simulink subsystem "station1"  (R2024b)
settings: Solver=VariableStepAuto  StartTime=0.0  StopTime=10.0  RelTol=1e-3
undefined symbols (not defined in the file): DiscIntNeverNeededParam, DPL1ph, h, Half, R3, ResistanceM, Rt4, simetran, Ts, Zm
libraries: fl_lib x215, ee_lib x97, nesl_utility x43, spsThreePhaseHarmonicFilterLib x21, simulink x7, spsThreePhaseSeriesRLCLoadLib x7, spsThreePhaseBreakerLib x7
(part 3 of 6)

== system station1/Filters 60Hz5 ==
  note: 60 Hz filters 4*150 Mvars @ 500 kV
  note: High-pass
      | damped filter
  note: Tuned filters
  note: Capacitor banks
  s : Inport
  11th 150 Mvar Q=100 : spsThreePhaseHarmonicFilterLib/Three-Phase Harmonic Filter  Commented=on  LConnTagsString=A|B|C  FilterType=Single-tuned  FilterConnection=Y (grounded)  ParNom=[500e3 60]  Qc=150e6/4  Fr=[11*60]  Frd=[11*60 13*60]  Q=100  Measurements=None
      settings: AttributesFormatString=\n
      settings: LibrarySourceBlock=|
      | sps_lib/Passives/Three-Phase
      | Harmonic Filter
  "13th 150 Mvar Q=100 " : spsThreePhaseHarmonicFilterLib/Three-Phase Harmonic Filter  Commented=on  LConnTagsString=A|B|C  FilterType=Single-tuned  FilterConnection=Y (grounded)  ParNom=[500e3 60]  Qc=150e6/4  Fr=[13*60]  Frd=[11*60 13*60]  Q=100  Measurements=None
      settings: AttributesFormatString=\n
      settings: LibrarySourceBlock=|
      | sps_lib/Passives/Three-Phase
      | Harmonic Filter
  150 Mvar : spsThreePhaseSeriesRLCLoadLib/Three-Phase Series RLC Load  Commented=on  LConnTagsString=A|B|C  Configuration=Y (grounded)  NominalVoltage=500e3  Vabc=[1e3 1e3 1e3]  Vabcp=[1e3 1e3 1e3]  NominalFrequency=60  UnbalancedPower=off  ActivePower=0  InductivePower=0  CapacitivePower=150e6/4  Pabc=[10e3 9e3 11e3]  QLabc=[100 90 110]  QCabc=[100 90 110]  Pabcp=[10e3 9e3 11e3]  QLabcp=[100 90 110]  QCabcp=[100 90 110]  Measurements=None  LoadType=constant Z
  24th 150 Mvar Q=3 : spsThreePhaseHarmonicFilterLib/Three-Phase Harmonic Filter  Commented=on  LConnTagsString=A|B|C  FilterType=High-pass  FilterConnection=Y (grounded)  ParNom=[500e3 60]  Qc=150e6/4  Fr=[24*60]  Frd=[11*60 13*60]  Q=3  Measurements=None
      settings: AttributesFormatString=\n
      settings: LibrarySourceBlock=|
      | sps_lib/Passives/Three-Phase
      | Harmonic Filter
  Circuit Breaker (Three-Phase) : ee_lib/Switches & Breakers/Circuit Breaker (Three-Phase)  R_closed=0.001 Ohm  G_open=1e-6 1/Ohm  threshold=0.5 V  breaker_behavior=ee.enum.switches.breakerBehavior.zeroCrossingEnable
      settings: InternalSimscapePortConfiguration="{\"Bottom\":[],\"Left\":[{\"id\":\"vT\",\"label\":\"vT\",\"type\":\"input\"},{\"id\":\"N1\",\"label\":\"~1\",\"type\":\"foundation.electrical.three_phase\"}],\"Right\":[{\"id\":\"N2\",\"label\":\"~2\",\"type\":\"foundation.electrical.three_phase\"}],\"Top\":[]}"
  Constant : Constant
  Electrical Reference : fl_lib/Electrical/Electrical Elements/Electrical Reference
  High-pass filter : Subsystem  mask(Three-Phase Harmonic Filter){FilterType=High-pass, FilterConnection=Y (grounded), ParNom=[500e3 60], Qc=150e6/4, Fr=[5*60], Frd=[24*60], Q=3}
      mask prompts: FilterType "Type of filter:"; FilterConnection "Filter connection:"; ParNom "Nominal L-L voltage and frequency  [Vn(Vrms) fn(Hz)]:"; Qc "Nominal reactive power (var):"; Fr "Tuning frequency (Hz)"; Frd "Tuning frequencies [ Fr1 (Hz)   Fr2 (Hz) ]"; Q "Quality factor (Q):"
      mask help:
      | Implements a three-phase harmonic filter.
      | The filter is built up from passive RLC components. Their values are computed using the specified  nominal reactive power, tuning frequency (ies) and quality factor.
      mask init: same as station1/Filters 60Hz1/High-pass filter
      mask Help: helpview(psbhelp);
      mask TypeOptions FilterType: Single-tuned | Double-tuned | High-pass | C-type High-pass
      mask Callback FilterType: %powericon('ThreePhaseHarmonicFilterCback',gcb);
      mask TypeOptions FilterConnection: Y (grounded) | Y (floating) | Y (neutral) | Delta
      mask Callback FilterConnection: %powericon('ThreePhaseHarmonicFilterCback',gcb);
      mask Display:
      | plot(12,0,88,95)
      | plot(C1_xo+cx0,C1_yo+cy0,C1_xo+cx1,C1_yo+cy1,C1_xo+cx2,C1_yo+cy2,C1_xo+cx3,C1_yo+cy3)
      | plot(L1_xo+lx0,L1_yo+ly0,L1_xo+lx1,L1_yo+ly1,L1_xo+lx2,L1_yo+ly2,L1_xo+lx3,L1_yo+ly3,L1_xo+lx4,L1_yo+ly4)
      | plot(R1_xo+rx0,R1_yo+ry0,R1_xo+rx1,R1_yo+ry1,R1_xo+rx2,R1_yo+ry2)
      | plot(C2_xo+cx0,C2_yo+cy0,C2_xo+cx1,C2_yo+cy1,C2_xo+cx2,C2_yo+cy2,C2_xo+cx3,C2_yo+cy3)
      | plot(L2_xo+lx0,L2_yo+ly0,L2_xo+lx1,L2_yo+ly1,L2_xo+lx2,L2_yo+ly2,L2_xo+lx3,L2_yo+ly3,L2_xo+lx4,L2_yo+ly4)
      | plot(s1x,s1y,s2x,s2y,s3x,s3y,s4x,s4y)
      | plot(g_xo+gx1,g_yo+gy1,g_xo+gx2,g_yo+gy2,g_xo+gx3,g_yo+gy3,g_xo+gx4,g_yo+gy4)
  Simulink-PS Converter : nesl_utility/Simulink-PS Converter  PhysicalDomain=network_engine_domain  SubClassName=ps_input  LeftPortType=input  RightPortType=output  PseudoPeriodic=off  Frequencies=[]  NoiseDistribution=none  NoiseParameters=[]  Unit=1  AffineConversion=off  FilteringAndDerivatives=provide  SimscapeFilterOrder=1  InputFilterTimeConstant=0.001  UdotUserProvided=0
  Sum : Sum  Inputs=|-+
  Three-Phase Breaker : spsThreePhaseBreakerLib/Three-Phase Breaker  Commented=on  InitialState=open  SwitchA=on  SwitchB=on  SwitchC=on  SwitchTimes=[1.5]  External=on  BreakerResistance=0.001  SnubberResistance=1e6  SnubberCapacitance=inf  Measurements=None
  Wye-Connected Load : ee_lib/Passive/RLC Assemblies/Wye-Connected Load  port_option=ee.enum.threePhasePort.composite  parameterization=ee.enum.rlc.parameterization.ratedpower  component_structure=ee.enum.rlc.structure.R  component_structure_PQ=ee.enum.rlc.structure.C  R=1 Ohm  L=1e-3 H  C=1e-6 F  VRated=500e3 V  FRated=60 Hz  P=1e3 W  Qpos=1e2 A*V  Qneg=-150e6/4 A*V  R_parasitic=1e-6 Ohm  G_parasitic=1e-6 1/Ohm  R_parasitic_PQ=0 Ohm  G_parasitic_PQ=1e-6 1/Ohm  Vmag0=500e3 V  Vang0=0 deg  Freq0=60 Hz  IL_specify=off  IL_priority=High  IL=[0, 0, 0] A  IL_nominal_specify=off  IL_nominal_value=1  IL_nominal_unit=A  VC_specify=off  VC_priority=High  VC=[0, 0, 0] V  VC_nominal_specify=off  VC_nominal_value=1  VC_nominal_unit=V
  tuned filter 11th : Subsystem  mask(Three-Phase Harmonic Filter){FilterType=Single-tuned, FilterConnection=Y (grounded), ParNom=[500e3 60], Qc=150e6/4, Fr=[5*60], Frd=[11*60], Q=100}
      mask prompts: FilterType "Type of filter:"; FilterConnection "Filter connection:"; ParNom "Nominal L-L voltage and frequency  [Vn(Vrms) fn(Hz)]:"; Qc "Nominal reactive power (var):"; Fr "Tuning frequency (Hz)"; Frd "Tuning frequencies [ Fr1 (Hz)   Fr2 (Hz) ]"; Q "Quality factor (Q):"
      mask help:
      | Implements a three-phase harmonic filter.
      | The filter is built up from passive RLC components. Their values are computed using the specified  nominal reactive power, tuning frequency (ies) and quality factor.
      mask init: same as station1/Filters 60Hz1/High-pass filter
      mask Help: helpview(psbhelp);
      mask TypeOptions FilterType: Single-tuned | Double-tuned | High-pass | C-type High-pass
      mask Callback FilterType: %powericon('ThreePhaseHarmonicFilterCback',gcb);
      mask TypeOptions FilterConnection: Y (grounded) | Y (floating) | Y (neutral) | Delta
      mask Callback FilterConnection: %powericon('ThreePhaseHarmonicFilterCback',gcb);
      mask Display:
      | plot(12,0,88,95)
      | plot(C1_xo+cx0,C1_yo+cy0,C1_xo+cx1,C1_yo+cy1,C1_xo+cx2,C1_yo+cy2,C1_xo+cx3,C1_yo+cy3)
      | plot(L1_xo+lx0,L1_yo+ly0,L1_xo+lx1,L1_yo+ly1,L1_xo+lx2,L1_yo+ly2,L1_xo+lx3,L1_yo+ly3,L1_xo+lx4,L1_yo+ly4)
      | plot(R1_xo+rx0,R1_yo+ry0,R1_xo+rx1,R1_yo+ry1,R1_xo+rx2,R1_yo+ry2)
      | plot(C2_xo+cx0,C2_yo+cy0,C2_xo+cx1,C2_yo+cy1,C2_xo+cx2,C2_yo+cy2,C2_xo+cx3,C2_yo+cy3)
      | plot(L2_xo+lx0,L2_yo+ly0,L2_xo+lx1,L2_yo+ly1,L2_xo+lx2,L2_yo+ly2,L2_xo+lx3,L2_yo+ly3,L2_xo+lx4,L2_yo+ly4)
      | plot(s1x,s1y,s2x,s2y,s3x,s3y,s4x,s4y)
      | plot(g_xo+gx1,g_yo+gy1,g_xo+gx2,g_yo+gy2,g_xo+gx3,g_yo+gy3,g_xo+gx4,g_yo+gy4)
  tuned filter 13th : Subsystem  mask(Three-Phase Harmonic Filter){FilterType=Single-tuned, FilterConnection=Y (grounded), ParNom=[500e3 60], Qc=150e6/4, Fr=[5*60], Frd=[13*60], Q=100}
      mask prompts: FilterType "Type of filter:"; FilterConnection "Filter connection:"; ParNom "Nominal L-L voltage and frequency  [Vn(Vrms) fn(Hz)]:"; Qc "Nominal reactive power (var):"; Fr "Tuning frequency (Hz)"; Frd "Tuning frequencies [ Fr1 (Hz)   Fr2 (Hz) ]"; Q "Quality factor (Q):"
      mask help:
      | Implements a three-phase harmonic filter.
      | The filter is built up from passive RLC components. Their values are computed using the specified  nominal reactive power, tuning frequency (ies) and quality factor.
      mask init: same as station1/Filters 60Hz1/High-pass filter
      mask Help: helpview(psbhelp);
      mask TypeOptions FilterType: Single-tuned | Double-tuned | High-pass | C-type High-pass
      mask Callback FilterType: %powericon('ThreePhaseHarmonicFilterCback',gcb);
      mask TypeOptions FilterConnection: Y (grounded) | Y (floating) | Y (neutral) | Delta
      mask Callback FilterConnection: %powericon('ThreePhaseHarmonicFilterCback',gcb);
      mask Display:
      | plot(12,0,88,95)
      | plot(C1_xo+cx0,C1_yo+cy0,C1_xo+cx1,C1_yo+cy1,C1_xo+cx2,C1_yo+cy2,C1_xo+cx3,C1_yo+cy3)
      | plot(L1_xo+lx0,L1_yo+ly0,L1_xo+lx1,L1_yo+ly1,L1_xo+lx2,L1_yo+ly2,L1_xo+lx3,L1_yo+ly3,L1_xo+lx4,L1_yo+ly4)
      | plot(R1_xo+rx0,R1_yo+ry0,R1_xo+rx1,R1_yo+ry1,R1_xo+rx2,R1_yo+ry2)
      | plot(C2_xo+cx0,C2_yo+cy0,C2_xo+cx1,C2_yo+cy1,C2_xo+cx2,C2_yo+cy2,C2_xo+cx3,C2_yo+cy3)
      | plot(L2_xo+lx0,L2_yo+ly0,L2_xo+lx1,L2_yo+ly1,L2_xo+lx2,L2_yo+ly2,L2_xo+lx3,L2_yo+ly3,L2_xo+lx4,L2_yo+ly4)
      | plot(s1x,s1y,s2x,s2y,s3x,s3y,s4x,s4y)
      | plot(g_xo+gx1,g_yo+gy1,g_xo+gx2,g_yo+gy2,g_xo+gx3,g_yo+gy3,g_xo+gx4,g_yo+gy4)
  abc : PMIOPort  Side=Right
  wires:
  s/1 -> Sum/1
  Constant/1 -> Sum/2
  Sum/1 -> Simulink-PS Converter/1
  connections:
  Three-Phase Breaker/LConn1 -- 150 Mvar/LConn1 -- 11th 150 Mvar Q=100/LConn1 -- "13th 150 Mvar Q=100 "/LConn1 -- 24th 150 Mvar Q=3/LConn1
  Three-Phase Breaker/LConn2 -- 150 Mvar/LConn2 -- 11th 150 Mvar Q=100/LConn2 -- "13th 150 Mvar Q=100 "/LConn2 -- 24th 150 Mvar Q=3/LConn2
  Three-Phase Breaker/LConn3 -- 150 Mvar/LConn3 -- 11th 150 Mvar Q=100/LConn3 -- "13th 150 Mvar Q=100 "/LConn3 -- 24th 150 Mvar Q=3/LConn3
  Electrical Reference/LConn1 -- Wye-Connected Load/RConn1
  Circuit Breaker (Three-Phase)/LConn2 -- tuned filter 13th/RConn1 -- Wye-Connected Load/LConn1 -- tuned filter 11th/RConn1 -- High-pass filter/RConn1
  Circuit Breaker (Three-Phase)/RConn1 -- abc/RConn1
  Simulink-PS Converter/RConn1 -- Circuit Breaker (Three-Phase)/LConn1

== system station1/Filters 60Hz6 ==
  note: Capacitor banks
  note: Tuned filters
  note: High-pass
      | damped filter
  note: 60 Hz filters 4*150 Mvars @ 500 kV
  s : Inport
  11th 150 Mvar Q=100 : spsThreePhaseHarmonicFilterLib/Three-Phase Harmonic Filter  Commented=on  LConnTagsString=A|B|C  FilterType=Single-tuned  FilterConnection=Y (grounded)  ParNom=[500e3 60]  Qc=150e6/4  Fr=[11*60]  Frd=[11*60 13*60]  Q=100  Measurements=None
      settings: AttributesFormatString=\n
      settings: LibrarySourceBlock=|
      | sps_lib/Passives/Three-Phase
      | Harmonic Filter
  "13th 150 Mvar Q=100 " : spsThreePhaseHarmonicFilterLib/Three-Phase Harmonic Filter  Commented=on  LConnTagsString=A|B|C  FilterType=Single-tuned  FilterConnection=Y (grounded)  ParNom=[500e3 60]  Qc=150e6/4  Fr=[13*60]  Frd=[11*60 13*60]  Q=100  Measurements=None
      settings: AttributesFormatString=\n
      settings: LibrarySourceBlock=|
      | sps_lib/Passives/Three-Phase
      | Harmonic Filter
  150 Mvar : spsThreePhaseSeriesRLCLoadLib/Three-Phase Series RLC Load  Commented=on  LConnTagsString=A|B|C  Configuration=Y (grounded)  NominalVoltage=500e3  Vabc=[1e3 1e3 1e3]  Vabcp=[1e3 1e3 1e3]  NominalFrequency=60  UnbalancedPower=off  ActivePower=0  InductivePower=0  CapacitivePower=150e6/4  Pabc=[10e3 9e3 11e3]  QLabc=[100 90 110]  QCabc=[100 90 110]  Pabcp=[10e3 9e3 11e3]  QLabcp=[100 90 110]  QCabcp=[100 90 110]  Measurements=None  LoadType=constant Z
  24th 150 Mvar Q=3 : spsThreePhaseHarmonicFilterLib/Three-Phase Harmonic Filter  Commented=on  LConnTagsString=A|B|C  FilterType=High-pass  FilterConnection=Y (grounded)  ParNom=[500e3 60]  Qc=150e6/4  Fr=[24*60]  Frd=[11*60 13*60]  Q=3  Measurements=None
      settings: AttributesFormatString=\n
      settings: LibrarySourceBlock=|
      | sps_lib/Passives/Three-Phase
      | Harmonic Filter
  Circuit Breaker (Three-Phase) : ee_lib/Switches & Breakers/Circuit Breaker (Three-Phase)  R_closed=0.001 Ohm  G_open=1e-6 1/Ohm  threshold=0.5 V  breaker_behavior=ee.enum.switches.breakerBehavior.zeroCrossingEnable
      settings: InternalSimscapePortConfiguration="{\"Bottom\":[],\"Left\":[{\"id\":\"vT\",\"label\":\"vT\",\"type\":\"input\"},{\"id\":\"N1\",\"label\":\"~1\",\"type\":\"foundation.electrical.three_phase\"}],\"Right\":[{\"id\":\"N2\",\"label\":\"~2\",\"type\":\"foundation.electrical.three_phase\"}],\"Top\":[]}"
  Constant : Constant
  Electrical Reference : fl_lib/Electrical/Electrical Elements/Electrical Reference
  High-pass filter : Subsystem  mask(Three-Phase Harmonic Filter){FilterType=High-pass, FilterConnection=Y (grounded), ParNom=[500e3 60], Qc=150e6/4, Fr=[5*60], Frd=[24*60], Q=3}
      mask prompts: FilterType "Type of filter:"; FilterConnection "Filter connection:"; ParNom "Nominal L-L voltage and frequency  [Vn(Vrms) fn(Hz)]:"; Qc "Nominal reactive power (var):"; Fr "Tuning frequency (Hz)"; Frd "Tuning frequencies [ Fr1 (Hz)   Fr2 (Hz) ]"; Q "Quality factor (Q):"
      mask help:
      | Implements a three-phase harmonic filter.
      | The filter is built up from passive RLC components. Their values are computed using the specified  nominal reactive power, tuning frequency (ies) and quality factor.
      mask init: same as station1/Filters 60Hz1/High-pass filter
      mask Help: helpview(psbhelp);
      mask TypeOptions FilterType: Single-tuned | Double-tuned | High-pass | C-type High-pass
      mask Callback FilterType: %powericon('ThreePhaseHarmonicFilterCback',gcb);
      mask TypeOptions FilterConnection: Y (grounded) | Y (floating) | Y (neutral) | Delta
      mask Callback FilterConnection: %powericon('ThreePhaseHarmonicFilterCback',gcb);
      mask Display:
      | plot(12,0,88,95)
      | plot(C1_xo+cx0,C1_yo+cy0,C1_xo+cx1,C1_yo+cy1,C1_xo+cx2,C1_yo+cy2,C1_xo+cx3,C1_yo+cy3)
      | plot(L1_xo+lx0,L1_yo+ly0,L1_xo+lx1,L1_yo+ly1,L1_xo+lx2,L1_yo+ly2,L1_xo+lx3,L1_yo+ly3,L1_xo+lx4,L1_yo+ly4)
      | plot(R1_xo+rx0,R1_yo+ry0,R1_xo+rx1,R1_yo+ry1,R1_xo+rx2,R1_yo+ry2)
      | plot(C2_xo+cx0,C2_yo+cy0,C2_xo+cx1,C2_yo+cy1,C2_xo+cx2,C2_yo+cy2,C2_xo+cx3,C2_yo+cy3)
      | plot(L2_xo+lx0,L2_yo+ly0,L2_xo+lx1,L2_yo+ly1,L2_xo+lx2,L2_yo+ly2,L2_xo+lx3,L2_yo+ly3,L2_xo+lx4,L2_yo+ly4)
      | plot(s1x,s1y,s2x,s2y,s3x,s3y,s4x,s4y)
      | plot(g_xo+gx1,g_yo+gy1,g_xo+gx2,g_yo+gy2,g_xo+gx3,g_yo+gy3,g_xo+gx4,g_yo+gy4)
  Simulink-PS Converter : nesl_utility/Simulink-PS Converter  PhysicalDomain=network_engine_domain  SubClassName=ps_input  LeftPortType=input  RightPortType=output  PseudoPeriodic=off  Frequencies=[]  NoiseDistribution=none  NoiseParameters=[]  Unit=1  AffineConversion=off  FilteringAndDerivatives=provide  SimscapeFilterOrder=1  InputFilterTimeConstant=0.001  UdotUserProvided=0
  Sum : Sum  Inputs=|-+
  Three-Phase Breaker : spsThreePhaseBreakerLib/Three-Phase Breaker  Commented=on  InitialState=open  SwitchA=on  SwitchB=on  SwitchC=on  SwitchTimes=[1.5]  External=on  BreakerResistance=0.001  SnubberResistance=1e6  SnubberCapacitance=inf  Measurements=None
  Wye-Connected Load : ee_lib/Passive/RLC Assemblies/Wye-Connected Load  port_option=ee.enum.threePhasePort.composite  parameterization=ee.enum.rlc.parameterization.ratedpower  component_structure=ee.enum.rlc.structure.R  component_structure_PQ=ee.enum.rlc.structure.C  R=1 Ohm  L=1e-3 H  C=1e-6 F  VRated=500e3 V  FRated=60 Hz  P=1e3 W  Qpos=1e2 A*V  Qneg=-150e6/4 A*V  R_parasitic=1e-6 Ohm  G_parasitic=1e-6 1/Ohm  R_parasitic_PQ=0 Ohm  G_parasitic_PQ=1e-6 1/Ohm  Vmag0=500e3 V  Vang0=0 deg  Freq0=60 Hz  IL_specify=off  IL_priority=High  IL=[0, 0, 0] A  IL_nominal_specify=off  IL_nominal_value=1  IL_nominal_unit=A  VC_specify=off  VC_priority=High  VC=[0, 0, 0] V  VC_nominal_specify=off  VC_nominal_value=1  VC_nominal_unit=V
  tuned filter 11th : Subsystem  mask(Three-Phase Harmonic Filter){FilterType=Single-tuned, FilterConnection=Y (grounded), ParNom=[500e3 60], Qc=150e6/4, Fr=[5*60], Frd=[11*60], Q=100}
      mask prompts: FilterType "Type of filter:"; FilterConnection "Filter connection:"; ParNom "Nominal L-L voltage and frequency  [Vn(Vrms) fn(Hz)]:"; Qc "Nominal reactive power (var):"; Fr "Tuning frequency (Hz)"; Frd "Tuning frequencies [ Fr1 (Hz)   Fr2 (Hz) ]"; Q "Quality factor (Q):"
      mask help:
      | Implements a three-phase harmonic filter.
      | The filter is built up from passive RLC components. Their values are computed using the specified  nominal reactive power, tuning frequency (ies) and quality factor.
      mask init: same as station1/Filters 60Hz1/High-pass filter
      mask Help: helpview(psbhelp);
      mask TypeOptions FilterType: Single-tuned | Double-tuned | High-pass | C-type High-pass
      mask Callback FilterType: %powericon('ThreePhaseHarmonicFilterCback',gcb);
      mask TypeOptions FilterConnection: Y (grounded) | Y (floating) | Y (neutral) | Delta
      mask Callback FilterConnection: %powericon('ThreePhaseHarmonicFilterCback',gcb);
      mask Display:
      | plot(12,0,88,95)
      | plot(C1_xo+cx0,C1_yo+cy0,C1_xo+cx1,C1_yo+cy1,C1_xo+cx2,C1_yo+cy2,C1_xo+cx3,C1_yo+cy3)
      | plot(L1_xo+lx0,L1_yo+ly0,L1_xo+lx1,L1_yo+ly1,L1_xo+lx2,L1_yo+ly2,L1_xo+lx3,L1_yo+ly3,L1_xo+lx4,L1_yo+ly4)
      | plot(R1_xo+rx0,R1_yo+ry0,R1_xo+rx1,R1_yo+ry1,R1_xo+rx2,R1_yo+ry2)
      | plot(C2_xo+cx0,C2_yo+cy0,C2_xo+cx1,C2_yo+cy1,C2_xo+cx2,C2_yo+cy2,C2_xo+cx3,C2_yo+cy3)
      | plot(L2_xo+lx0,L2_yo+ly0,L2_xo+lx1,L2_yo+ly1,L2_xo+lx2,L2_yo+ly2,L2_xo+lx3,L2_yo+ly3,L2_xo+lx4,L2_yo+ly4)
      | plot(s1x,s1y,s2x,s2y,s3x,s3y,s4x,s4y)
      | plot(g_xo+gx1,g_yo+gy1,g_xo+gx2,g_yo+gy2,g_xo+gx3,g_yo+gy3,g_xo+gx4,g_yo+gy4)
  tuned filter 13th : Subsystem  mask(Three-Phase Harmonic Filter){FilterType=Single-tuned, FilterConnection=Y (grounded), ParNom=[500e3 60], Qc=150e6/4, Fr=[5*60], Frd=[13*60], Q=100}
      mask prompts: FilterType "Type of filter:"; FilterConnection "Filter connection:"; ParNom "Nominal L-L voltage and frequency  [Vn(Vrms) fn(Hz)]:"; Qc "Nominal reactive power (var):"; Fr "Tuning frequency (Hz)"; Frd "Tuning frequencies [ Fr1 (Hz)   Fr2 (Hz) ]"; Q "Quality factor (Q):"
      mask help:
      | Implements a three-phase harmonic filter.
      | The filter is built up from passive RLC components. Their values are computed using the specified  nominal reactive power, tuning frequency (ies) and quality factor.
      mask init: same as station1/Filters 60Hz1/High-pass filter
      mask Help: helpview(psbhelp);
      mask TypeOptions FilterType: Single-tuned | Double-tuned | High-pass | C-type High-pass
      mask Callback FilterType: %powericon('ThreePhaseHarmonicFilterCback',gcb);
      mask TypeOptions FilterConnection: Y (grounded) | Y (floating) | Y (neutral) | Delta
      mask Callback FilterConnection: %powericon('ThreePhaseHarmonicFilterCback',gcb);
      mask Display:
      | plot(12,0,88,95)
      | plot(C1_xo+cx0,C1_yo+cy0,C1_xo+cx1,C1_yo+cy1,C1_xo+cx2,C1_yo+cy2,C1_xo+cx3,C1_yo+cy3)
      | plot(L1_xo+lx0,L1_yo+ly0,L1_xo+lx1,L1_yo+ly1,L1_xo+lx2,L1_yo+ly2,L1_xo+lx3,L1_yo+ly3,L1_xo+lx4,L1_yo+ly4)
      | plot(R1_xo+rx0,R1_yo+ry0,R1_xo+rx1,R1_yo+ry1,R1_xo+rx2,R1_yo+ry2)
      | plot(C2_xo+cx0,C2_yo+cy0,C2_xo+cx1,C2_yo+cy1,C2_xo+cx2,C2_yo+cy2,C2_xo+cx3,C2_yo+cy3)
      | plot(L2_xo+lx0,L2_yo+ly0,L2_xo+lx1,L2_yo+ly1,L2_xo+lx2,L2_yo+ly2,L2_xo+lx3,L2_yo+ly3,L2_xo+lx4,L2_yo+ly4)
      | plot(s1x,s1y,s2x,s2y,s3x,s3y,s4x,s4y)
      | plot(g_xo+gx1,g_yo+gy1,g_xo+gx2,g_yo+gy2,g_xo+gx3,g_yo+gy3,g_xo+gx4,g_yo+gy4)
  abc : PMIOPort  Side=Right
  wires:
  Sum/1 -> Simulink-PS Converter/1
  Constant/1 -> Sum/2
  s/1 -> Sum/1
  connections:
  Simulink-PS Converter/RConn1 -- Circuit Breaker (Three-Phase)/LConn1
  Circuit Breaker (Three-Phase)/RConn1 -- abc/RConn1
  High-pass filter/RConn1 -- tuned filter 11th/RConn1 -- Wye-Connected Load/LConn1 -- tuned filter 13th/RConn1 -- Circuit Breaker (Three-Phase)/LConn2
  Electrical Reference/LConn1 -- Wye-Connected Load/RConn1
  24th 150 Mvar Q=3/LConn3 -- "13th 150 Mvar Q=100 "/LConn3 -- 11th 150 Mvar Q=100/LConn3 -- 150 Mvar/LConn3 -- Three-Phase Breaker/LConn3
  24th 150 Mvar Q=3/LConn2 -- "13th 150 Mvar Q=100 "/LConn2 -- 11th 150 Mvar Q=100/LConn2 -- 150 Mvar/LConn2 -- Three-Phase Breaker/LConn2
  24th 150 Mvar Q=3/LConn1 -- "13th 150 Mvar Q=100 "/LConn1 -- 11th 150 Mvar Q=100/LConn1 -- 150 Mvar/LConn1 -- Three-Phase Breaker/LConn1

== system station1/Filters 60Hz7 ==
  note: 60 Hz filters 4*150 Mvars @ 500 kV
  note: High-pass
      | damped filter
  note: Tuned filters
  note: Capacitor banks
  s : Inport
  11th 150 Mvar Q=100 : spsThreePhaseHarmonicFilterLib/Three-Phase Harmonic Filter  Commented=on  LConnTagsString=A|B|C  FilterType=Single-tuned  FilterConnection=Y (grounded)  ParNom=[500e3 60]  Qc=150e6/4  Fr=[11*60]  Frd=[11*60 13*60]  Q=100  Measurements=None
      settings: AttributesFormatString=\n
      settings: LibrarySourceBlock=|
      | sps_lib/Passives/Three-Phase
      | Harmonic Filter
  "13th 150 Mvar Q=100 " : spsThreePhaseHarmonicFilterLib/Three-Phase Harmonic Filter  Commented=on  LConnTagsString=A|B|C  FilterType=Single-tuned  FilterConnection=Y (grounded)  ParNom=[500e3 60]  Qc=150e6/4  Fr=[13*60]  Frd=[11*60 13*60]  Q=100  Measurements=None
      settings: AttributesFormatString=\n
      settings: LibrarySourceBlock=|
      | sps_lib/Passives/Three-Phase
      | Harmonic Filter
  150 Mvar : spsThreePhaseSeriesRLCLoadLib/Three-Phase Series RLC Load  Commented=on  LConnTagsString=A|B|C  Configuration=Y (grounded)  NominalVoltage=500e3  Vabc=[1e3 1e3 1e3]  Vabcp=[1e3 1e3 1e3]  NominalFrequency=60  UnbalancedPower=off  ActivePower=0  InductivePower=0  CapacitivePower=150e6/4  Pabc=[10e3 9e3 11e3]  QLabc=[100 90 110]  QCabc=[100 90 110]  Pabcp=[10e3 9e3 11e3]  QLabcp=[100 90 110]  QCabcp=[100 90 110]  Measurements=None  LoadType=constant Z
  24th 150 Mvar Q=3 : spsThreePhaseHarmonicFilterLib/Three-Phase Harmonic Filter  Commented=on  LConnTagsString=A|B|C  FilterType=High-pass  FilterConnection=Y (grounded)  ParNom=[500e3 60]  Qc=150e6/4  Fr=[24*60]  Frd=[11*60 13*60]  Q=3  Measurements=None
      settings: AttributesFormatString=\n
      settings: LibrarySourceBlock=|
      | sps_lib/Passives/Three-Phase
      | Harmonic Filter
  Circuit Breaker (Three-Phase) : ee_lib/Switches & Breakers/Circuit Breaker (Three-Phase)  R_closed=0.001 Ohm  G_open=1e-6 1/Ohm  threshold=0.5 V  breaker_behavior=ee.enum.switches.breakerBehavior.zeroCrossingEnable
      settings: InternalSimscapePortConfiguration="{\"Bottom\":[],\"Left\":[{\"id\":\"vT\",\"label\":\"vT\",\"type\":\"input\"},{\"id\":\"N1\",\"label\":\"~1\",\"type\":\"foundation.electrical.three_phase\"}],\"Right\":[{\"id\":\"N2\",\"label\":\"~2\",\"type\":\"foundation.electrical.three_phase\"}],\"Top\":[]}"
  Constant : Constant
  Electrical Reference : fl_lib/Electrical/Electrical Elements/Electrical Reference
  High-pass filter : Subsystem  mask(Three-Phase Harmonic Filter){FilterType=High-pass, FilterConnection=Y (grounded), ParNom=[500e3 60], Qc=150e6/4, Fr=[5*60], Frd=[24*60], Q=3}
      mask prompts: FilterType "Type of filter:"; FilterConnection "Filter connection:"; ParNom "Nominal L-L voltage and frequency  [Vn(Vrms) fn(Hz)]:"; Qc "Nominal reactive power (var):"; Fr "Tuning frequency (Hz)"; Frd "Tuning frequencies [ Fr1 (Hz)   Fr2 (Hz) ]"; Q "Quality factor (Q):"
      mask help:
      | Implements a three-phase harmonic filter.
      | The filter is built up from passive RLC components. Their values are computed using the specified  nominal reactive power, tuning frequency (ies) and quality factor.
      mask init: same as station1/Filters 60Hz1/High-pass filter
      mask Help: helpview(psbhelp);
      mask TypeOptions FilterType: Single-tuned | Double-tuned | High-pass | C-type High-pass
      mask Callback FilterType: %powericon('ThreePhaseHarmonicFilterCback',gcb);
      mask TypeOptions FilterConnection: Y (grounded) | Y (floating) | Y (neutral) | Delta
      mask Callback FilterConnection: %powericon('ThreePhaseHarmonicFilterCback',gcb);
      mask Display:
      | plot(12,0,88,95)
      | plot(C1_xo+cx0,C1_yo+cy0,C1_xo+cx1,C1_yo+cy1,C1_xo+cx2,C1_yo+cy2,C1_xo+cx3,C1_yo+cy3)
      | plot(L1_xo+lx0,L1_yo+ly0,L1_xo+lx1,L1_yo+ly1,L1_xo+lx2,L1_yo+ly2,L1_xo+lx3,L1_yo+ly3,L1_xo+lx4,L1_yo+ly4)
      | plot(R1_xo+rx0,R1_yo+ry0,R1_xo+rx1,R1_yo+ry1,R1_xo+rx2,R1_yo+ry2)
      | plot(C2_xo+cx0,C2_yo+cy0,C2_xo+cx1,C2_yo+cy1,C2_xo+cx2,C2_yo+cy2,C2_xo+cx3,C2_yo+cy3)
      | plot(L2_xo+lx0,L2_yo+ly0,L2_xo+lx1,L2_yo+ly1,L2_xo+lx2,L2_yo+ly2,L2_xo+lx3,L2_yo+ly3,L2_xo+lx4,L2_yo+ly4)
      | plot(s1x,s1y,s2x,s2y,s3x,s3y,s4x,s4y)
      | plot(g_xo+gx1,g_yo+gy1,g_xo+gx2,g_yo+gy2,g_xo+gx3,g_yo+gy3,g_xo+gx4,g_yo+gy4)
  Simulink-PS Converter : nesl_utility/Simulink-PS Converter  PhysicalDomain=network_engine_domain  SubClassName=ps_input  LeftPortType=input  RightPortType=output  PseudoPeriodic=off  Frequencies=[]  NoiseDistribution=none  NoiseParameters=[]  Unit=1  AffineConversion=off  FilteringAndDerivatives=provide  SimscapeFilterOrder=1  InputFilterTimeConstant=0.001  UdotUserProvided=0
  Sum : Sum  Inputs=|-+
  Three-Phase Breaker : spsThreePhaseBreakerLib/Three-Phase Breaker  Commented=on  InitialState=open  SwitchA=on  SwitchB=on  SwitchC=on  SwitchTimes=[1.5]  External=on  BreakerResistance=0.001  SnubberResistance=1e6  SnubberCapacitance=inf  Measurements=None
  Wye-Connected Load : ee_lib/Passive/RLC Assemblies/Wye-Connected Load  port_option=ee.enum.threePhasePort.composite  parameterization=ee.enum.rlc.parameterization.ratedpower  component_structure=ee.enum.rlc.structure.R  component_structure_PQ=ee.enum.rlc.structure.C  R=1 Ohm  L=1e-3 H  C=1e-6 F  VRated=500e3 V  FRated=60 Hz  P=1e3 W  Qpos=1e2 A*V  Qneg=-150e6/4 A*V  R_parasitic=1e-6 Ohm  G_parasitic=1e-6 1/Ohm  R_parasitic_PQ=0 Ohm  G_parasitic_PQ=1e-6 1/Ohm  Vmag0=500e3 V  Vang0=0 deg  Freq0=60 Hz  IL_specify=off  IL_priority=High  IL=[0, 0, 0] A  IL_nominal_specify=off  IL_nominal_value=1  IL_nominal_unit=A  VC_specify=off  VC_priority=High  VC=[0, 0, 0] V  VC_nominal_specify=off  VC_nominal_value=1  VC_nominal_unit=V
  tuned filter 11th : Subsystem  mask(Three-Phase Harmonic Filter){FilterType=Single-tuned, FilterConnection=Y (grounded), ParNom=[500e3 60], Qc=150e6/4, Fr=[5*60], Frd=[11*60], Q=100}
      mask prompts: FilterType "Type of filter:"; FilterConnection "Filter connection:"; ParNom "Nominal L-L voltage and frequency  [Vn(Vrms) fn(Hz)]:"; Qc "Nominal reactive power (var):"; Fr "Tuning frequency (Hz)"; Frd "Tuning frequencies [ Fr1 (Hz)   Fr2 (Hz) ]"; Q "Quality factor (Q):"
      mask help:
      | Implements a three-phase harmonic filter.
      | The filter is built up from passive RLC components. Their values are computed using the specified  nominal reactive power, tuning frequency (ies) and quality factor.
      mask init: same as station1/Filters 60Hz1/High-pass filter
      mask Help: helpview(psbhelp);
      mask TypeOptions FilterType: Single-tuned | Double-tuned | High-pass | C-type High-pass
      mask Callback FilterType: %powericon('ThreePhaseHarmonicFilterCback',gcb);
      mask TypeOptions FilterConnection: Y (grounded) | Y (floating) | Y (neutral) | Delta
      mask Callback FilterConnection: %powericon('ThreePhaseHarmonicFilterCback',gcb);
      mask Display:
      | plot(12,0,88,95)
      | plot(C1_xo+cx0,C1_yo+cy0,C1_xo+cx1,C1_yo+cy1,C1_xo+cx2,C1_yo+cy2,C1_xo+cx3,C1_yo+cy3)
      | plot(L1_xo+lx0,L1_yo+ly0,L1_xo+lx1,L1_yo+ly1,L1_xo+lx2,L1_yo+ly2,L1_xo+lx3,L1_yo+ly3,L1_xo+lx4,L1_yo+ly4)
      | plot(R1_xo+rx0,R1_yo+ry0,R1_xo+rx1,R1_yo+ry1,R1_xo+rx2,R1_yo+ry2)
      | plot(C2_xo+cx0,C2_yo+cy0,C2_xo+cx1,C2_yo+cy1,C2_xo+cx2,C2_yo+cy2,C2_xo+cx3,C2_yo+cy3)
      | plot(L2_xo+lx0,L2_yo+ly0,L2_xo+lx1,L2_yo+ly1,L2_xo+lx2,L2_yo+ly2,L2_xo+lx3,L2_yo+ly3,L2_xo+lx4,L2_yo+ly4)
      | plot(s1x,s1y,s2x,s2y,s3x,s3y,s4x,s4y)
      | plot(g_xo+gx1,g_yo+gy1,g_xo+gx2,g_yo+gy2,g_xo+gx3,g_yo+gy3,g_xo+gx4,g_yo+gy4)
  tuned filter 13th : Subsystem  mask(Three-Phase Harmonic Filter){FilterType=Single-tuned, FilterConnection=Y (grounded), ParNom=[500e3 60], Qc=150e6/4, Fr=[5*60], Frd=[13*60], Q=100}
      mask prompts: FilterType "Type of filter:"; FilterConnection "Filter connection:"; ParNom "Nominal L-L voltage and frequency  [Vn(Vrms) fn(Hz)]:"; Qc "Nominal reactive power (var):"; Fr "Tuning frequency (Hz)"; Frd "Tuning frequencies [ Fr1 (Hz)   Fr2 (Hz) ]"; Q "Quality factor (Q):"
      mask help:
      | Implements a three-phase harmonic filter.
      | The filter is built up from passive RLC components. Their values are computed using the specified  nominal reactive power, tuning frequency (ies) and quality factor.
      mask init: same as station1/Filters 60Hz1/High-pass filter
      mask Help: helpview(psbhelp);
      mask TypeOptions FilterType: Single-tuned | Double-tuned | High-pass | C-type High-pass
      mask Callback FilterType: %powericon('ThreePhaseHarmonicFilterCback',gcb);
      mask TypeOptions FilterConnection: Y (grounded) | Y (floating) | Y (neutral) | Delta
      mask Callback FilterConnection: %powericon('ThreePhaseHarmonicFilterCback',gcb);
      mask Display:
      | plot(12,0,88,95)
      | plot(C1_xo+cx0,C1_yo+cy0,C1_xo+cx1,C1_yo+cy1,C1_xo+cx2,C1_yo+cy2,C1_xo+cx3,C1_yo+cy3)
      | plot(L1_xo+lx0,L1_yo+ly0,L1_xo+lx1,L1_yo+ly1,L1_xo+lx2,L1_yo+ly2,L1_xo+lx3,L1_yo+ly3,L1_xo+lx4,L1_yo+ly4)
      | plot(R1_xo+rx0,R1_yo+ry0,R1_xo+rx1,R1_yo+ry1,R1_xo+rx2,R1_yo+ry2)
      | plot(C2_xo+cx0,C2_yo+cy0,C2_xo+cx1,C2_yo+cy1,C2_xo+cx2,C2_yo+cy2,C2_xo+cx3,C2_yo+cy3)
      | plot(L2_xo+lx0,L2_yo+ly0,L2_xo+lx1,L2_yo+ly1,L2_xo+lx2,L2_yo+ly2,L2_xo+lx3,L2_yo+ly3,L2_xo+lx4,L2_yo+ly4)
      | plot(s1x,s1y,s2x,s2y,s3x,s3y,s4x,s4y)
      | plot(g_xo+gx1,g_yo+gy1,g_xo+gx2,g_yo+gy2,g_xo+gx3,g_yo+gy3,g_xo+gx4,g_yo+gy4)
  abc : PMIOPort  Side=Right
  wires:
  s/1 -> Sum/1
  Constant/1 -> Sum/2
  Sum/1 -> Simulink-PS Converter/1
  connections:
  Three-Phase Breaker/LConn1 -- 150 Mvar/LConn1 -- 11th 150 Mvar Q=100/LConn1 -- "13th 150 Mvar Q=100 "/LConn1 -- 24th 150 Mvar Q=3/LConn1
  Three-Phase Breaker/LConn2 -- 150 Mvar/LConn2 -- 11th 150 Mvar Q=100/LConn2 -- "13th 150 Mvar Q=100 "/LConn2 -- 24th 150 Mvar Q=3/LConn2
  Three-Phase Breaker/LConn3 -- 150 Mvar/LConn3 -- 11th 150 Mvar Q=100/LConn3 -- "13th 150 Mvar Q=100 "/LConn3 -- 24th 150 Mvar Q=3/LConn3
  Electrical Reference/LConn1 -- Wye-Connected Load/RConn1
  Circuit Breaker (Three-Phase)/LConn2 -- tuned filter 13th/RConn1 -- Wye-Connected Load/LConn1 -- tuned filter 11th/RConn1 -- High-pass filter/RConn1
  Circuit Breaker (Three-Phase)/RConn1 -- abc/RConn1
  Simulink-PS Converter/RConn1 -- Circuit Breaker (Three-Phase)/LConn1

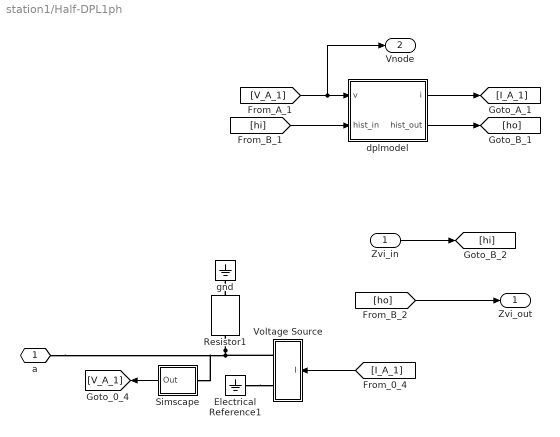
== system station1/Half-DPL1ph ==
  Zvi_in : Inport
  Electrical Reference1 : fl_lib/Electrical/Electrical Elements/Electrical Reference
  Resistor1 : ee_lib/Passive/Resistor  R=ResistanceM(1,1) Ohm  enable_R_tol=ee.enum.toleranceApplication.none  R_tol=5  tol_distribution=ee.enum.toleranceDistribution.uniform  nSigma=4  enable_operating_limits=ee.enum.enable.no  operating_limit_action=ee.enum.passive.reportOpLim.warn  power_rating=1 W  max_working_voltage=100 V  noise_mode=ee.enum.sources.noise.Disabled  Tdevice=25 degC  sample_time=1e-3 s  repeatability=ee.enum.ic.repeatability.notRepeatable  user_seed=0  auto_seed=3499211588  fault_action=simscape.enum.assert.action.none  t_fault=1 s  power_derating_T1=70 degC  power_derating_T2=155 degC  operating_temperature_range_vec=[-50, 150] degC  alpha=3.93e-3 1/K  Tmeas=25 degC  thermal_mass=100 J/K  temperature_specify=off  temperature_priority=High  temperature=298.15 K  temperature_nominal_specify=off  temperature_nominal_value=1  temperature_nominal_unit=K
  Simscape : Subsystem
      mask Display: disp('V')
  Voltage Source : Subsystem
  dplmodel : Subsystem
  gnd : fl_lib/Electrical/Electrical Elements/Electrical Reference
  a : PMIOPort  Side=Left
  Zvi_out : Outport  VectorParamsAs1DForOutWhenUnconnected=off
  Vnode : Outport  Port=2  VectorParamsAs1DForOutWhenUnconnected=off
  wires:
  [I_A_1] -> Voltage Source/1(I)
  Simscape/1(Out) -> [V_A_1]
  dplmodel/2(hist_out) -> [ho]
  [hi] -> dplmodel/2(hist_in)
  Zvi_in/1 -> [hi]
  [V_A_1] -> dplmodel/1(v), Vnode/1
  dplmodel/1(i) -> [I_A_1]
  [ho] -> Zvi_out/1
  connections:
  Electrical Reference1/LConn1 -- Voltage Source/RConn2
  Resistor1/LConn1 -- gnd/LConn1
  Resistor1/RConn1 -- Voltage Source/RConn1 -- Simscape/LConn1 -- a/RConn1
